simulink model "FlybackConverter"  (R2018b)
settings: Solver=VariableStepAuto  StartTime=0.0  StopTime=0.1  MaxStep=1e-4  RelTol=1e-4  EnableMultiTasking=on
libraries: powerlib x21, pePwmGenerator x1
Description:
  | Copyright 2008-2018 The MathWorks, Inc.
settings Model: Creator=MathWorks  LastModifiedBy=MONSTER
settings SolverCC: SolverResetMethod=Robust
settings DataIOCC: ReturnWorkspaceOutputs=on
settings OptimizationCC: LifeSpan=inf
settings DebuggingCC: ReadBeforeWriteMsg=DisableAll  WriteAfterWriteMsg=DisableAll  WriteAfterReadMsg=DisableAll  MultiTaskDSMMsg=none  LibraryContextMissingDiagnostic=none  SFUnexpectedBacktrackingDiag=warning  SFNoUnconditionalDefaultTransitionDiag=warning  SFExecutionAtInitializationDiag=none
settings ModelReferenceCC: UpdateModelReferenceTargets=IfOutOfDate
settings SFSimCC: SFSimEcho=off  SimUseLocalCustomCode=off
settings RTWCC: RTWUseLocalCustomCode=off
settings CodeAppCC: StateflowObjectComments=on
settings GRTTargetCC: TargetLangStandard=C89/C90 (ANSI)  GeneratePreprocessorConditionals=Disable all
settings ConfigComp: CovMetricSettings=dw  CovHtmlReporting=on  CovSaveCumulativeToWorkspaceVar=on  CovSaveSingleToWorkspaceVar=on  CovExternalEMLEnable=off
settings SimscapeCC: SimscapeNormalizeSystem=off  SimscapeNominalValues={1, 'bar'; 1, 'cm^3/s'; 1, 'bar*kg/s'; 1, 'kJ/kg'; 1, 'kW'; }

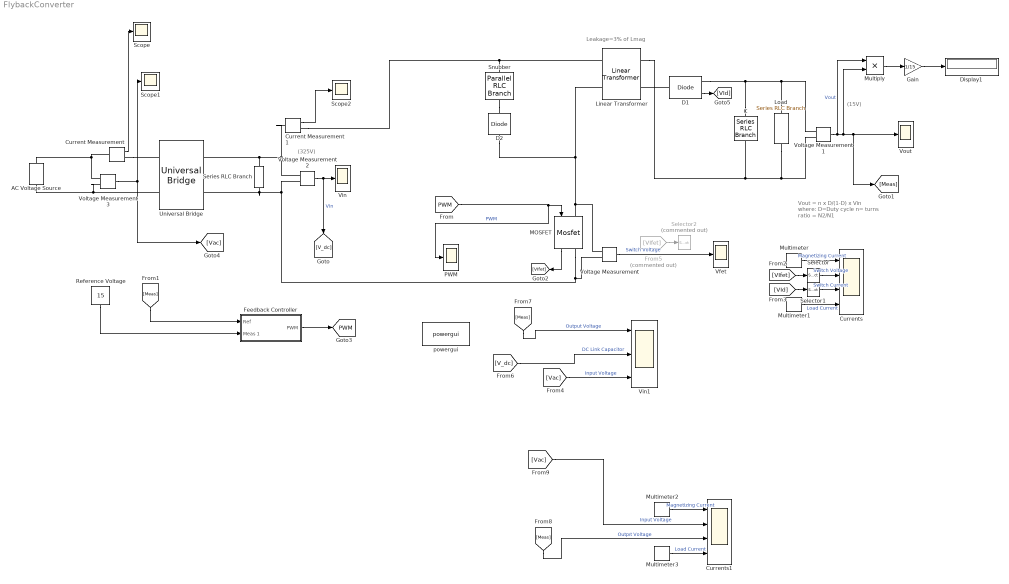
== system FlybackConverter ==
  note: (15V)
  note: Leakage=3% of Lmag
  note: Vout = n x D/(1-D) x Vin
      | where: D=Duty cycle
      | n= turns ratio = N2/N1
  note: (325V)
  AC Voltage Source : powerlib/Electrical Sources/AC Voltage Source  Amplitude=325  Phase=0  Frequency=50  SampleTime=0  Measurements=None  BusType=swing  Pref=10e3  Qref=0  Qmin=-inf  Qmax=+inf
      settings: SourceProductName=Simscape Electrical
  C : powerlib/Elements/Series RLC Branch  LConnTagsString=__new0  RConnTagsString=__new0  BranchType=C  Resistance=1e-4  Inductance=200e-6  SetiL0=off  InitialCurrent=0  Capacitance=2e-3  Setx0=off  InitialVoltage=0  Measurements=None
      settings: SourceProductName=Simscape Electrical
  Current Measurement : powerlib/Measurements/Current Measurement  PhasorSimulation=off  OutputType=Complex  PSBequivalent=0
      settings: SourceProductName=Simscape Electrical
  Current Measurement1 : powerlib/Measurements/Current Measurement  PhasorSimulation=off  OutputType=Complex  PSBequivalent=0
      settings: SourceProductName=Simscape Electrical
  Currents : Scope  NumInputPorts=4
  Currents1 : Scope  NumInputPorts=4
  D1 : powerlib/Power Electronics/Diode  Ron=1e-3  Lon=0  Vf=0  IC=0  UseSnubber=off  Rs=inf  Cs=0  Measurements=on
      settings: SourceProductName=Simscape Electrical
  D2 : powerlib/Power Electronics/Diode  Ron=1e-3  Lon=0  Vf=0  IC=0  UseSnubber=off  Rs=inf  Cs=0  Measurements=off
      settings: SourceProductName=Simscape Electrical
  Display1 : Display
  Feedback Controller : Subsystem
  From5 : From  Commented=on  GotoTag=VIfet
  Gain : Gain  Gain=1/15
  Linear Transformer : powerlib/Elements/Linear Transformer  UNITS=SI  NominalPower=[ 25 100e3 ]  winding1=[300 0 0]  winding2=[20 0 0]  ThreeWindings=off  winding3=[3.15e+05 3.969e+07 6316.9]  RmLm=[1e4 1000e-6]  Measurements=Magnetization current  DataType=on
      settings: SourceProductName=Simscape Electrical
  Load : powerlib/Elements/Series RLC Branch  LConnTagsString=__new0  RConnTagsString=__new0  BranchType=R  Resistance=15  Inductance=200e-6  SetiL0=off  InitialCurrent=0  Capacitance=400e-6  Setx0=off  InitialVoltage=0  Measurements=Branch current
      settings: SourceProductName=Simscape Electrical
  MOSFET : powerlib/Power Electronics/Mosfet  Ron=1e-3  Lon=0  Rd=1e-3  Vfd=0  IC=0  Rs=1e6  Cs=inf  Measurements=on
      settings: SourceProductName=Simscape Electrical
  Multimeter : powerlib/Measurements/Multimeter  PhasorSimulation=off  OutputType=Complex  sel=3  L=4  Gain=1  yselected={'Imag: Linear Transformer'};  PSBOutputType=1  PSBequivalent=0  AxesSetting=[0,0.1,-100,100]  Display=0  SavedBlockNames=-11
      settings: SourceProductName=Simscape Electrical
  Multimeter1 : powerlib/Measurements/Multimeter  PhasorSimulation=off  OutputType=Complex  sel=1  L=4  Gain=1  yselected={'Ib: Load'};  PSBOutputType=1  PSBequivalent=0  AxesSetting=[0,0.1,-100,100]  Display=0  SavedBlockNames=-11
      settings: SourceProductName=Simscape Electrical
  Multimeter2 : powerlib/Measurements/Multimeter  PhasorSimulation=off  OutputType=Complex  sel=3  L=4  Gain=1  yselected={'Imag: Linear Transformer'};  PSBOutputType=1  PSBequivalent=0  AxesSetting=[0,0.1,-100,100]  Display=0  SavedBlockNames=-11
      settings: SourceProductName=Simscape Electrical
  Multimeter3 : powerlib/Measurements/Multimeter  PhasorSimulation=off  OutputType=Complex  sel=1  L=4  Gain=1  yselected={'Ib: Load'};  PSBOutputType=1  PSBequivalent=0  AxesSetting=[0,0.1,-100,100]  Display=0  SavedBlockNames=-11
      settings: SourceProductName=Simscape Electrical
  Multiply : Product
  PWM : Scope
  "Reference Voltage " : Constant  Value=15
  Scope : Scope
  Scope1 : Scope
  Scope2 : Scope
  Selector : Selector  InputPortWidth=2  IndexOptions=Index vector (dialog)  Indices=1  OutputSizes=1
  Selector1 : Selector  InputPortWidth=2  IndexOptions=Index vector (dialog)  Indices=1  OutputSizes=1
  Selector2 : Selector  Commented=on  InputPortWidth=2  IndexOptions=Index vector (dialog)  Indices=2  OutputSizes=1
  Series RLC Branch : powerlib/Elements/Series RLC Branch  LConnTagsString=__new0  RConnTagsString=__new0  BranchType=C  Resistance=1  Inductance=1e-3  SetiL0=off  InitialCurrent=0  Capacitance=800e-6  Setx0=off  InitialVoltage=0  Measurements=None
      settings: SourceProductName=Simscape Electrical
  Snubber : powerlib/Elements/Parallel RLC Branch  LConnTagsString=a  RConnTagsString=__new0  BranchType=RC  Resistance=10e3  Inductance=1e-3  SetiL0=off  InitialCurrent=0  Capacitance=89e-9  Setx0=off  InitialVoltage=0  Measurements=None
      settings: SourceProductName=Simscape Electrical
  Universal Bridge : powerlib/Power Electronics/Universal Bridge  Arms=2  SnubberResistance=1e5  SnubberCapacitance=inf  Device=Diodes  Ron=1e-3  Lon=0  ForwardVoltages="[  0  0  ]"  ForwardVoltage=0  GTOparameters=[ 10e-6 , 20e-6 ]  IGBTparameters=[ 1e-6 , 2e-6 ]  Measurements=None  Measurements_2=None  converterType=Rectifier
      settings: SourceProductName=Simscape Electrical
  Vfet : Scope
  Vin : Scope
  Vin1 : Scope  NumInputPorts=3
  Voltage Measurement{,1..3} (4 alike) : powerlib/Measurements/Voltage Measurement  PhasorSimulation=off  OutputType=Complex  PSBequivalent=0
      settings: SourceProductName=Simscape Electrical
  Vout : Scope
  powergui : powerlib/powergui  Priority=1  SimulationMode=Continuous  SampleTime=50e-6  frequency=60  Iterations=50  frequencyindice=50  Pbase=100e6  ErrMax=1e-4  UnitsV=kV  UnitsW=MW  buscounter=0  FunctionMessages=off  echomessages=off  EnableUseOfTLC=off  CurrentSourceSwitches=off  DisableSnubberDevices=off  DisableRonSwitches=off  DisableVfSwitches=off  DisplayEquations=off  SolverType=Tustin/Backward Euler (TBE)  Interpol=off  ExternalGateDelay=off  methode=off  Ts=100  x0status=blocks  SPID=on  SwTol=0  HookPort=off  RestoreLinks=warning  ResistiveCurrentMeasurement=off  Frange=[0:2:500]  Ylog=off  Xlog=on  ShowGrid=off  save=off  variable=ZData  structure=0  ZoomFFT=off  StartTime=0.0  cycles=1  DisplayStyle=1  fundamental=60  FreqAxis=off  MaxFrequency=1000  frequencyindicesteady=1  RmsSteady=1  display=off
      settings: SourceProductName=Simscape Electrical
  tag scope: PWM=global
  wires:
  Voltage Measurement1/1 -> Multiply/1, Multiply/2, [Meas], Vout/1  "Vout"
  MOSFET/1 -> [VIfet]
  D1/1 -> [VId]
  Multimeter/1 -> Currents/1  "Magnetizing Current"
  Selector/1 -> Currents/2  "Switch Voltage"
  [VIfet] -> Selector/1
  Selector1/1 -> Currents/3  "Switch Current"
  [VId] -> Selector1/1
  Multimeter1/1 -> Currents/4  "Load Current"
  From5/1 -> Selector2/1
  Voltage Measurement2/1 -> Vin/1, [V_dc]  "Vin"
  [PWM] -> PWM/1, MOSFET/1  "PWM"
  "Reference Voltage "/1 -> Feedback Controller/2(Meas 1)
  [Meas] -> Feedback Controller/1("Ref ")
  Voltage Measurement3/1 -> Scope1/1, [Vac]
  [Vac] -> Vin1/3  "Input Voltage"
  [V_dc] -> Vin1/2  "DC Link Capacitor"
  [Meas] -> Vin1/1  "Output Voltage"
  Feedback Controller/1("PWM ") -> [PWM]
  Voltage Measurement/1 -> Vfet/1  "Switch Voltage"
  Multimeter3/1 -> Currents1/4  "Load Current"
  Multimeter2/1 -> Currents1/1  "Magnetizing Current"
  [Meas] -> Currents1/3  "Outpıt Voltage"
  [Vac] -> Currents1/2  "Input Voltage"
  Multiply/1 -> Gain/1
  Gain/1 -> Display1/1
  Current Measurement/1 -> Scope/1
  Current Measurement1/1 -> Scope2/1
  connections:
  C/LConn1 -- Voltage Measurement1/LConn1 -- Load/LConn1 -- D1/RConn1
  Load/RConn1 -- Voltage Measurement1/LConn2 -- Linear Transformer/RConn1 -- C/RConn1
  Linear Transformer/LConn2 -- D2/LConn1 -- Voltage Measurement/LConn1 -- MOSFET/LConn1
  D1/LConn1 -- Linear Transformer/RConn2
  Snubber/RConn1 -- D2/RConn1
  AC Voltage Source/LConn1 -- Voltage Measurement3/LConn2 -- Universal Bridge/LConn2
  Voltage Measurement3/LConn1 -- Current Measurement/LConn1 -- AC Voltage Source/RConn1
  Snubber/LConn1 -- Current Measurement1/RConn1 -- Linear Transformer/LConn1
  Series RLC Branch/RConn1 -- Voltage Measurement/LConn2 -- MOSFET/RConn1 -- Voltage Measurement2/LConn2 -- Universal Bridge/RConn2
  Current Measurement/RConn1 -- Universal Bridge/LConn1
  Voltage Measurement2/LConn1 -- Current Measurement1/LConn1 -- Universal Bridge/RConn1 -- Series RLC Branch/LConn1

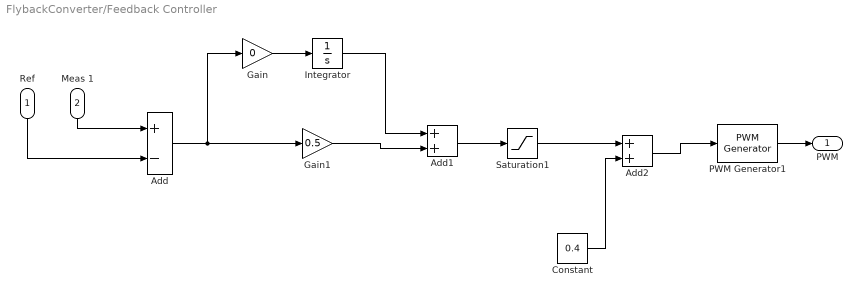
== system FlybackConverter/Feedback Controller ==
  "Ref " : Inport
  Meas 1 : Inport  Port=2
  Add : Sum  Inputs=+-
  Add1 : Sum
  Add2 : Sum
  Constant : Constant  Value=0.4
  Gain : Gain  Gain=0
  Gain1 : Gain  Gain=0.5
  Integrator : Integrator
  PWM Generator1 : pePwmGenerator/PWM Generator  CarrCount=Up  Tper=1e-6  Ts=1e-7
  Saturation1 : Saturate  UpperLimit=0.3  LowerLimit=-0.39
  "PWM " : Outport
  wires:
  "Ref "/1 -> Add/2
  Meas 1/1 -> Add/1
  Add/1 -> Gain1/1, Gain/1
  Add1/1 -> Saturation1/1
  PWM Generator1/1 -> "PWM "/1
  Gain/1 -> Integrator/1
  Integrator/1 -> Add1/1
  Gain1/1 -> Add1/2
  Saturation1/1 -> Add2/1
  Constant/1 -> Add2/2
  Add2/1 -> PWM Generator1/1
